simulink model "Complete_System"  (R2018b)
settings: Solver=ode4  StartTime=0.0  StopTime=5  FixedStep=Step_Size  RelTol=1e-3  EnableMultiTasking=on
InitFcn:
  | clc ;
  | clear all ;
  | close all ;
  | Missile_Data ;
  | Sim_Parameters ;
undefined symbols (not defined in the file): D, Tbl_ALPHAT, Tbl_CL_ALPHAT, Tbl_CL_DEL_R, Tbl_CL_P, Tbl_CM_0, Tbl_CM_DEL_P, Tbl_CM_PHIT, Tbl_CM_Q, Tbl_CN_DEL_Y, Tbl_CN_PHIT, Tbl_CN_R, Tbl_CX_0, Tbl_CX_ALPHAT, Tbl_CX_DEL_EFF, Tbl_CY_DEL_Y, Tbl_CY_PHIT, Tbl_CZ_0, Tbl_CZ_DEL_P, Tbl_CZ_PHIT, Tbl_MACH, XCG, XREF
libraries: simulink_extras x4, aerolibtransform2 x3
settings Model: Creator=e803534  LastModifiedBy=auten
settings OptimizationCC: LifeSpan=inf
settings DebuggingCC: UnconnectedInputMsg=none  UnconnectedOutputMsg=none  UnconnectedLineMsg=none  SFUnexpectedBacktrackingDiag=warning  SFNoUnconditionalDefaultTransitionDiag=warning
settings SFSimCC: SimUseLocalCustomCode=off
settings RTWCC: RTWUseLocalCustomCode=off
settings CodeAppCC: StateflowObjectComments=on
settings GRTTargetCC: TargetLangStandard=C89/C90 (ANSI)  GeneratePreprocessorConditionals=Disable all
settings ConfigComp: CovMetricSettings=dw  CovHtmlReporting=on  CovSaveCumulativeToWorkspaceVar=on  CovSaveSingleToWorkspaceVar=on  CovExternalEMLEnable=off

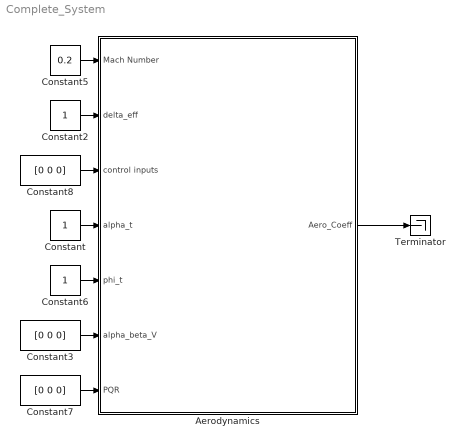
== system Complete_System ==
  Aerodynamics : Subsystem
  Constant : Constant
  Constant2 : Constant
  Constant3 : Constant  Value=[0 0 0]
  Constant5 : Constant  Value=0.2
  Constant6 : Constant
  Constant7 : Constant  Value=[0 0 0]
  Constant8 : Constant  Value=[0 0 0]
  Terminator : Terminator
  wires:
  Constant6/1 -> Aerodynamics/5(phi_t)
  Constant5/1 -> Aerodynamics/1(Mach Number)
  Constant2/1 -> Aerodynamics/2(delta_eff)
  Constant7/1 -> Aerodynamics/7(PQR)
  Constant/1 -> Aerodynamics/4(alpha_t)
  Constant8/1 -> Aerodynamics/3(control inputs)
  Constant3/1 -> Aerodynamics/6(alpha_beta_V)
  Aerodynamics/1(Aero_Coeff) -> Terminator/1

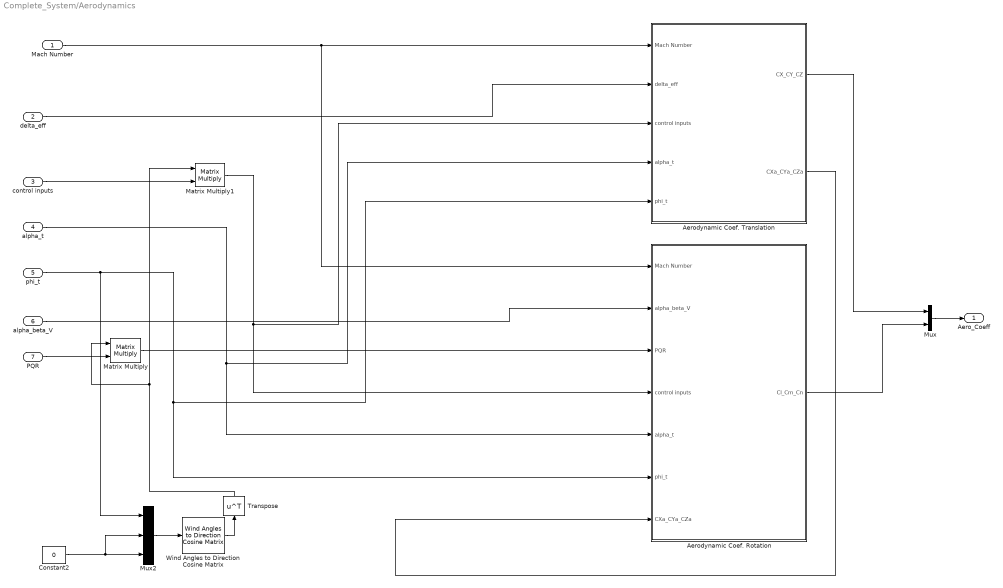
== system Complete_System/Aerodynamics ==
  Mach Number : Inport
  delta_eff : Inport  Port=2
  control inputs : Inport  Port=3
  alpha_t : Inport  Port=4
  phi_t : Inport  Port=5
  alpha_beta_V : Inport  Port=6
  PQR : Inport  Port=7
  Aerodynamic Coef. Rotation : Subsystem
  Aerodynamic Coef. Translation : Subsystem
  Constant2 : Constant  Value=0
  Matrix Multiply : Product  Multiplication=Matrix(*)
  Matrix Multiply1 : Product  Multiplication=Matrix(*)
  Mux : Mux  Inputs=2
  Mux2 : Mux  Inputs=3
  Transpose : Math  Operator=transpose  SaturateOnIntegerOverflow=on
  Wind Angles to Direction Cosine Matrix : aerolibtransform2/Wind Angles to  Direction Cosine Matrix
      settings: SourceProductName=Aerospace Blockset  SourceProductBaseCode=AE
  Aero_Coeff : Outport
  wires:
  Aerodynamic Coef. Translation/2(CXa_CYa_CZa) -> Aerodynamic Coef. Rotation/7(CXa_CYa_CZa)
  Mach Number/1 -> Aerodynamic Coef. Rotation/1(Mach Number), Aerodynamic Coef. Translation/1(Mach Number)
  delta_eff/1 -> Aerodynamic Coef. Translation/2(delta_eff)
  Matrix Multiply1/1 -> Aerodynamic Coef. Rotation/4(control inputs), Aerodynamic Coef. Translation/3(control inputs)
  alpha_beta_V/1 -> Aerodynamic Coef. Rotation/2(alpha_beta_V)
  Matrix Multiply/1 -> Aerodynamic Coef. Rotation/3(PQR)
  Aerodynamic Coef. Translation/1(CX_CY_CZ) -> Mux/1
  Aerodynamic Coef. Rotation/1(Cl_Cm_Cn) -> Mux/2
  Mux/1 -> Aero_Coeff/1
  alpha_t/1 -> Aerodynamic Coef. Rotation/5(alpha_t), Aerodynamic Coef. Translation/4(alpha_t)
  phi_t/1 -> Mux2/1, Aerodynamic Coef. Translation/5(phi_t), Aerodynamic Coef. Rotation/6(phi_t)
  Mux2/1 -> Wind Angles to Direction Cosine Matrix/1
  Constant2/1 -> Mux2/2, Mux2/3
  control inputs/1 -> Matrix Multiply1/2
  Wind Angles to Direction Cosine Matrix/1 -> Transpose/1
  PQR/1 -> Matrix Multiply/2
  Transpose/1 -> Matrix Multiply/1, Matrix Multiply1/1

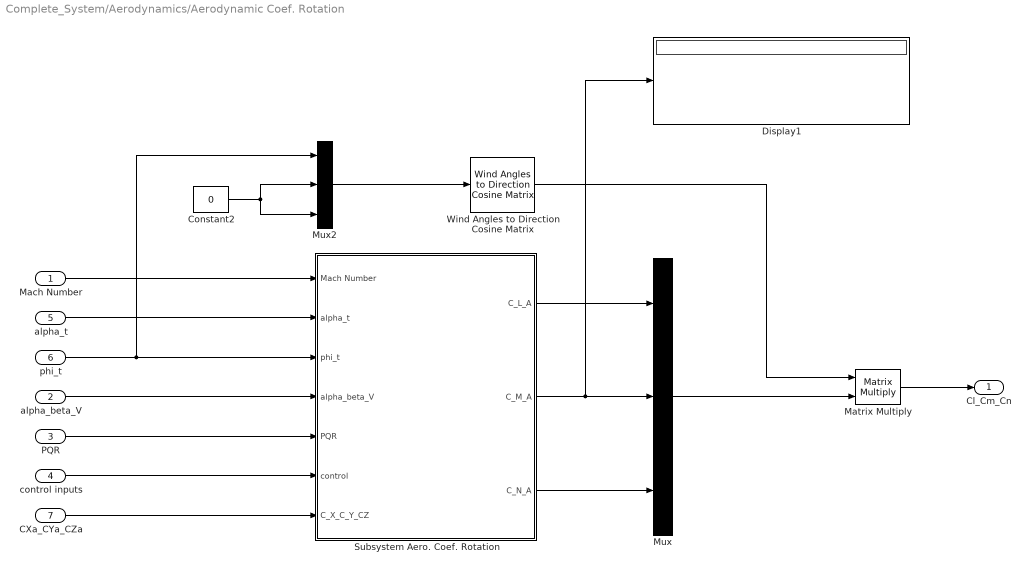
== system Complete_System/Aerodynamics/Aerodynamic Coef. Rotation ==
  Mach Number : Inport
  alpha_beta_V : Inport  Port=2
  PQR : Inport  Port=3
  control inputs : Inport  Port=4
  alpha_t : Inport  Port=5
  phi_t : Inport  Port=6
  CXa_CYa_CZa : Inport  Port=7
  Constant2 : Constant  Value=0
  Display1 : Display
  Matrix Multiply : Product  Multiplication=Matrix(*)
  Mux : Mux  Inputs=3
  Mux2 : Mux  Inputs=3
  Subsystem Aero. Coef. Rotation : Subsystem
  Wind Angles to Direction Cosine Matrix : aerolibtransform2/Wind Angles to  Direction Cosine Matrix
      settings: SourceProductName=Aerospace Blockset  SourceProductBaseCode=AE
  Cl_Cm_Cn : Outport
  wires:
  Mux/1 -> Matrix Multiply/2
  Matrix Multiply/1 -> Cl_Cm_Cn/1
  Mach Number/1 -> Subsystem Aero. Coef. Rotation/1(Mach Number)
  alpha_beta_V/1 -> Subsystem Aero. Coef. Rotation/4(alpha_beta_V)
  PQR/1 -> Subsystem Aero. Coef. Rotation/5(PQR)
  control inputs/1 -> Subsystem Aero. Coef. Rotation/6(control)
  alpha_t/1 -> Subsystem Aero. Coef. Rotation/2(alpha_t)
  phi_t/1 -> Mux2/1, Subsystem Aero. Coef. Rotation/3(phi_t)
  CXa_CYa_CZa/1 -> Subsystem Aero. Coef. Rotation/7(C_X_C_Y_CZ)
  Mux2/1 -> Wind Angles to Direction Cosine Matrix/1
  Constant2/1 -> Mux2/2, Mux2/3
  Wind Angles to Direction Cosine Matrix/1 -> Matrix Multiply/1
  Subsystem Aero. Coef. Rotation/1(C_L_A) -> Mux/1
  Subsystem Aero. Coef. Rotation/2(C_M_A) -> Display1/1, Mux/2
  Subsystem Aero. Coef. Rotation/3(C_N_A) -> Mux/3

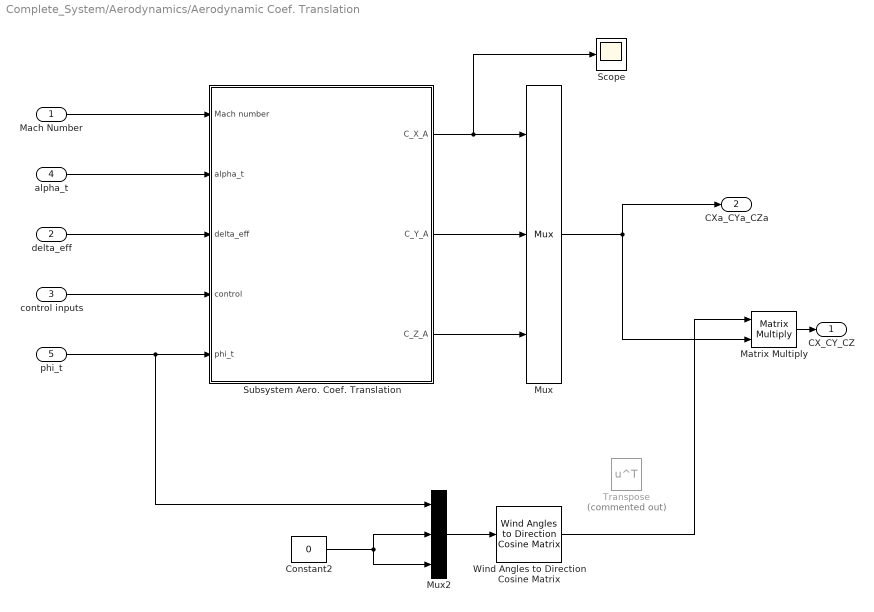
== system Complete_System/Aerodynamics/Aerodynamic Coef. Translation ==
  Mach Number : Inport
  delta_eff : Inport  Port=2
  control inputs : Inport  Port=3
  alpha_t : Inport  Port=4
  phi_t : Inport  Port=5
  Constant2 : Constant  Value=0
  Matrix Multiply : Product  Multiplication=Matrix(*)
  Mux : Mux  Inputs=3
  Mux2 : Mux  Inputs=3
  Scope : Scope
  Subsystem Aero. Coef. Translation : Subsystem
  Transpose : Math  Commented=on  Operator=transpose  SaturateOnIntegerOverflow=on
  Wind Angles to Direction Cosine Matrix : aerolibtransform2/Wind Angles to  Direction Cosine Matrix
      settings: SourceProductName=Aerospace Blockset  SourceProductBaseCode=AE
  CX_CY_CZ : Outport
  CXa_CYa_CZa : Outport  Port=2
  wires:
  Mux/1 -> Matrix Multiply/2, CXa_CYa_CZa/1
  Matrix Multiply/1 -> CX_CY_CZ/1
  Mux2/1 -> Wind Angles to Direction Cosine Matrix/1
  phi_t/1 -> Mux2/1, Subsystem Aero. Coef. Translation/5(phi_t)
  Constant2/1 -> Mux2/2, Mux2/3
  Mach Number/1 -> Subsystem Aero. Coef. Translation/1(Mach number)
  control inputs/1 -> Subsystem Aero. Coef. Translation/4(control)
  alpha_t/1 -> Subsystem Aero. Coef. Translation/2(alpha_t)
  delta_eff/1 -> Subsystem Aero. Coef. Translation/3(delta_eff)
  Subsystem Aero. Coef. Translation/1(C_X_A) -> Scope/1, Mux/1
  Subsystem Aero. Coef. Translation/2(C_Y_A) -> Mux/2
  Subsystem Aero. Coef. Translation/3(C_Z_A) -> Mux/3
  Wind Angles to Direction Cosine Matrix/1 -> Matrix Multiply/1

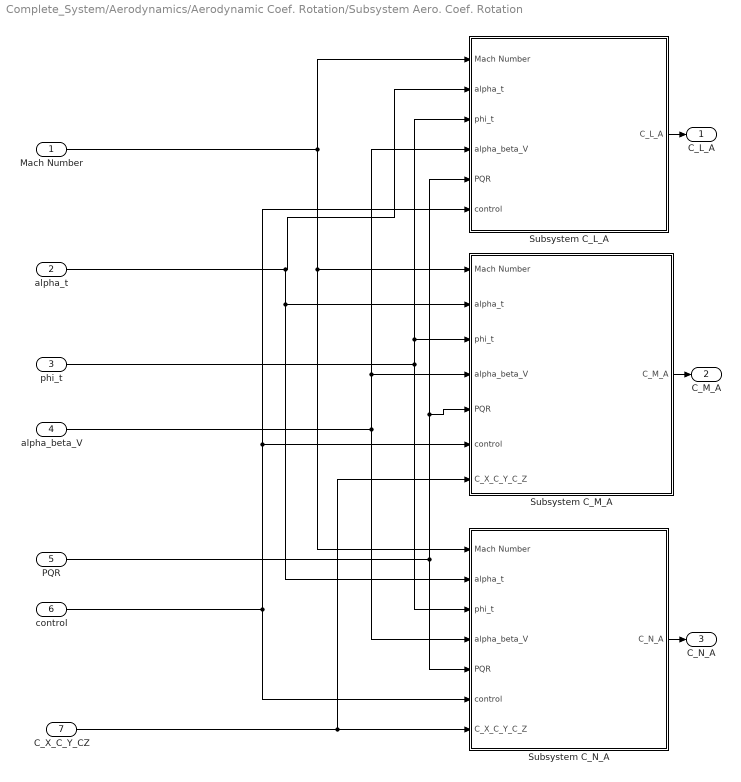
== system Complete_System/Aerodynamics/Aerodynamic Coef. Rotation/Subsystem Aero. Coef. Rotation ==
  Mach Number : Inport
  alpha_t : Inport  Port=2
  phi_t : Inport  Port=3
  alpha_beta_V : Inport  Port=4
  PQR : Inport  Port=5
  control : Inport  Port=6
  C_X_C_Y_CZ : Inport  Port=7
  "Subsystem C_L_A " : Subsystem
  "Subsystem C_M_A " : Subsystem
  Subsystem C_N_A : Subsystem
  C_L_A : Outport
  C_M_A : Outport  Port=2
  C_N_A : Outport  Port=3
  wires:
  "Subsystem C_M_A "/1(C_M_A) -> C_M_A/1
  "Subsystem C_L_A "/1(C_L_A) -> C_L_A/1
  Subsystem C_N_A/1(C_N_A) -> C_N_A/1
  Mach Number/1 -> "Subsystem C_L_A "/1(Mach Number), "Subsystem C_M_A "/1(Mach Number), Subsystem C_N_A/1(Mach Number)
  alpha_t/1 -> Subsystem C_N_A/2(alpha_t), "Subsystem C_M_A "/2(alpha_t), "Subsystem C_L_A "/2(alpha_t)
  phi_t/1 -> Subsystem C_N_A/3(phi_t), "Subsystem C_M_A "/3(phi_t), "Subsystem C_L_A "/3(phi_t)
  alpha_beta_V/1 -> "Subsystem C_L_A "/4(alpha_beta_V), "Subsystem C_M_A "/4(alpha_beta_V), Subsystem C_N_A/4(alpha_beta_V)
  PQR/1 -> "Subsystem C_M_A "/5(PQR), "Subsystem C_L_A "/5(PQR), Subsystem C_N_A/5(PQR)
  control/1 -> "Subsystem C_M_A "/6(control), "Subsystem C_L_A "/6(control), Subsystem C_N_A/6(control)
  C_X_C_Y_CZ/1 -> "Subsystem C_M_A "/7(C_X_C_Y_C_Z), Subsystem C_N_A/7(C_X_C_Y_C_Z)

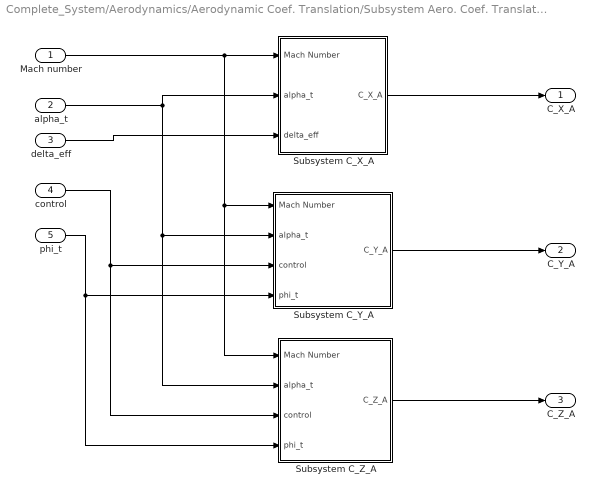
== system Complete_System/Aerodynamics/Aerodynamic Coef. Translation/Subsystem Aero. Coef. Translation ==
  Mach number : Inport
  alpha_t : Inport  Port=2
  delta_eff : Inport  Port=3
  control : Inport  Port=4
  phi_t : Inport  Port=5
  Subsystem C_X_A : Subsystem
  Subsystem C_Y_A : Subsystem
  Subsystem C_Z_A : Subsystem
  C_X_A : Outport
  C_Y_A : Outport  Port=2
  C_Z_A : Outport  Port=3
  wires:
  Subsystem C_X_A/1(C_X_A) -> C_X_A/1
  Subsystem C_Y_A/1(C_Y_A) -> C_Y_A/1
  Subsystem C_Z_A/1(C_Z_A) -> C_Z_A/1
  Mach number/1 -> Subsystem C_Z_A/1(Mach Number), Subsystem C_Y_A/1(Mach Number), Subsystem C_X_A/1(Mach Number)
  alpha_t/1 -> Subsystem C_Z_A/2(alpha_t), Subsystem C_Y_A/2(alpha_t), Subsystem C_X_A/2(alpha_t)
  delta_eff/1 -> Subsystem C_X_A/3(delta_eff)
  control/1 -> Subsystem C_Z_A/3(control), Subsystem C_Y_A/3(control)
  phi_t/1 -> Subsystem C_Z_A/4(phi_t), Subsystem C_Y_A/4(phi_t)

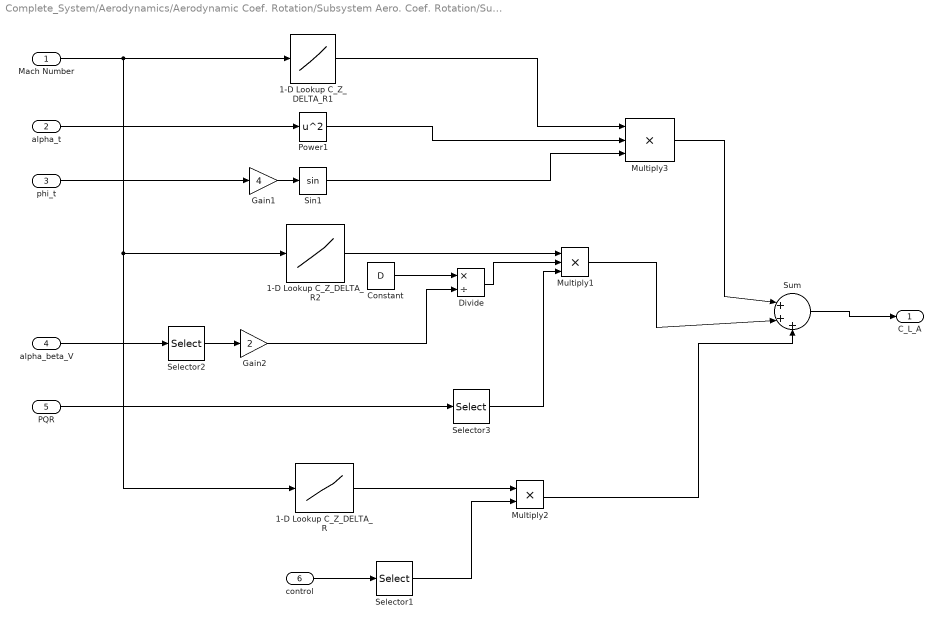
== system Complete_System/Aerodynamics/Aerodynamic Coef. Rotation/Subsystem Aero. Coef. Rotation/Subsystem C_L_A  ==
  Mach Number : Inport
  alpha_t : Inport  Port=2
  phi_t : Inport  Port=3
  alpha_beta_V : Inport  Port=4
  PQR : Inport  Port=5
  control : Inport  Port=6
  1-D Lookup C_Z_DELTA_R : Lookup_n-D  NumberOfTableDimensions=1  BreakpointsForDimension1=Tbl_MACH  Table=Tbl_CL_DEL_R  InternalRulePriority=Speed  RndMeth=Simplest  InputSameDT=on
  1-D Lookup C_Z_DELTA_R1 : Lookup_n-D  NumberOfTableDimensions=1  BreakpointsForDimension1=Tbl_MACH  Table=Tbl_CL_ALPHAT  InternalRulePriority=Speed  RndMeth=Simplest  InputSameDT=on
  1-D Lookup C_Z_DELTA_R2 : Lookup_n-D  NumberOfTableDimensions=1  BreakpointsForDimension1=Tbl_MACH  Table=Tbl_CL_P  InternalRulePriority=Speed  RndMeth=Simplest  InputSameDT=on
  Constant : Constant  Value=D
  Divide : Product  Inputs=*/
  Gain1 : Gain  Gain=4
  Gain2 : Gain  Gain=2
  Multiply1 : Product  Inputs=3
  Multiply2 : Product
  Multiply3 : Product  Inputs=3
  Power1 : Math  Operator=square  SaturateOnIntegerOverflow=on
  Selector1 : Selector  InputPortWidth=3  IndexOptions=Index vector (dialog)  Indices=[1]  OutputSizes=1
  Selector2 : Selector  InputPortWidth=3  IndexOptions=Index vector (dialog)  Indices=[3]  OutputSizes=1
  Selector3 : Selector  InputPortWidth=3  IndexOptions=Index vector (dialog)  Indices=[1]  OutputSizes=1
  Sin1 : Trigonometry
  Sum : Sum  Inputs=|+++
  C_L_A : Outport
  wires:
  1-D Lookup C_Z_DELTA_R1/1 -> Multiply3/1
  alpha_t/1 -> Power1/1
  Sum/1 -> C_L_A/1
  Mach Number/1 -> 1-D Lookup C_Z_DELTA_R/1, 1-D Lookup C_Z_DELTA_R2/1, 1-D Lookup C_Z_DELTA_R1/1
  1-D Lookup C_Z_DELTA_R2/1 -> Multiply1/1
  1-D Lookup C_Z_DELTA_R/1 -> Multiply2/1
  Multiply2/1 -> Sum/3
  Power1/1 -> Multiply3/2
  Sin1/1 -> Multiply3/3
  phi_t/1 -> Gain1/1
  Gain1/1 -> Sin1/1
  alpha_beta_V/1 -> Selector2/1
  Multiply3/1 -> Sum/1
  Multiply1/1 -> Sum/2
  Constant/1 -> Divide/1
  Selector2/1 -> Gain2/1
  Gain2/1 -> Divide/2
  Divide/1 -> Multiply1/2
  PQR/1 -> Selector3/1
  Selector3/1 -> Multiply1/3
  control/1 -> Selector1/1
  Selector1/1 -> Multiply2/2

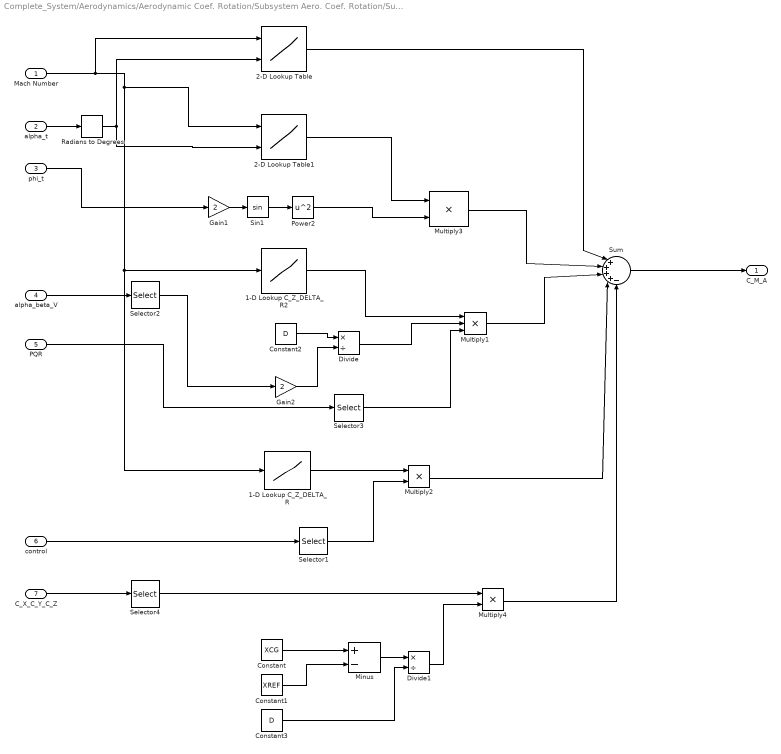
== system Complete_System/Aerodynamics/Aerodynamic Coef. Rotation/Subsystem Aero. Coef. Rotation/Subsystem C_M_A  ==
  Mach Number : Inport
  alpha_t : Inport  Port=2
  phi_t : Inport  Port=3
  alpha_beta_V : Inport  Port=4
  PQR : Inport  Port=5
  control : Inport  Port=6
  C_X_C_Y_C_Z : Inport  Port=7
  1-D Lookup C_Z_DELTA_R : Lookup_n-D  NumberOfTableDimensions=1  BreakpointsForDimension1=Tbl_MACH  Table=Tbl_CM_DEL_P  InternalRulePriority=Speed  RndMeth=Simplest  InputSameDT=on
  1-D Lookup C_Z_DELTA_R2 : Lookup_n-D  NumberOfTableDimensions=1  BreakpointsForDimension1=Tbl_MACH  Table=Tbl_CM_Q  DiagnosticForOutOfRangeInput=Warning  InternalRulePriority=Speed  RndMeth=Simplest  InputSameDT=on
  2-D Lookup Table : Lookup_n-D  BreakpointsForDimension1=Tbl_MACH  BreakpointsForDimension2=Tbl_ALPHAT  Table=Tbl_CM_0  DiagnosticForOutOfRangeInput=Warning  InternalRulePriority=Speed  RndMeth=Simplest  InputSameDT=on
  2-D Lookup Table1 : Lookup_n-D  BreakpointsForDimension1=Tbl_MACH  BreakpointsForDimension2=Tbl_ALPHAT  Table=Tbl_CM_PHIT  InternalRulePriority=Speed  RndMeth=Simplest  InputSameDT=on
  Constant : Constant  Value=XCG
  Constant1 : Constant  Value=XREF
  Constant2 : Constant  Value=D
  Constant3 : Constant  Value=D
  Divide : Product  Inputs=*/
  Divide1 : Product  Inputs=*/
  Gain1 : Gain  Gain=2
  Gain2 : Gain  Gain=2
  Minus : Sum  Inputs=+-
  Multiply1 : Product  Inputs=3
  Multiply2 : Product
  Multiply3 : Product
  Multiply4 : Product
  Power2 : Math  Operator=square  SaturateOnIntegerOverflow=on
  Radians to Degrees : simulink_extras/Transformations/Radians to Degrees
  Selector1 : Selector  InputPortWidth=3  IndexOptions=Index vector (dialog)  Indices=[2]  OutputSizes=1
  Selector2 : Selector  InputPortWidth=3  IndexOptions=Index vector (dialog)  Indices=[3]  OutputSizes=1
  Selector3 : Selector  InputPortWidth=3  IndexOptions=Index vector (dialog)  Indices=[2]  OutputSizes=1
  Selector4 : Selector  InputPortWidth=3  IndexOptions=Index vector (dialog)  Indices=[3]  OutputSizes=1
  Sin1 : Trigonometry
  Sum : Sum  Inputs=|++++-
  C_M_A : Outport
  wires:
  2-D Lookup Table/1 -> Sum/1
  Mach Number/1 -> 2-D Lookup Table/1, 2-D Lookup Table1/1, 1-D Lookup C_Z_DELTA_R/1, 1-D Lookup C_Z_DELTA_R2/1
  1-D Lookup C_Z_DELTA_R2/1 -> Multiply1/1
  1-D Lookup C_Z_DELTA_R/1 -> Multiply2/1
  Multiply2/1 -> Sum/4
  Sin1/1 -> Power2/1
  phi_t/1 -> Gain1/1
  Gain1/1 -> Sin1/1
  alpha_beta_V/1 -> Selector2/1
  Selector2/1 -> Gain2/1
  Gain2/1 -> Divide/2
  Divide/1 -> Multiply1/2
  PQR/1 -> Selector3/1
  Selector3/1 -> Multiply1/3
  control/1 -> Selector1/1
  Selector1/1 -> Multiply2/2
  2-D Lookup Table1/1 -> Multiply3/1
  Power2/1 -> Multiply3/2
  C_X_C_Y_C_Z/1 -> Selector4/1
  Constant/1 -> Minus/1
  Constant1/1 -> Minus/2
  Constant2/1 -> Divide/1
  Minus/1 -> Divide1/1
  Constant3/1 -> Divide1/2
  Selector4/1 -> Multiply4/1
  Divide1/1 -> Multiply4/2
  Multiply4/1 -> Sum/5
  Multiply1/1 -> Sum/3
  Multiply3/1 -> Sum/2
  alpha_t/1 -> Radians to Degrees/1
  Radians to Degrees/1 -> 2-D Lookup Table1/2, 2-D Lookup Table/2
  Sum/1 -> C_M_A/1

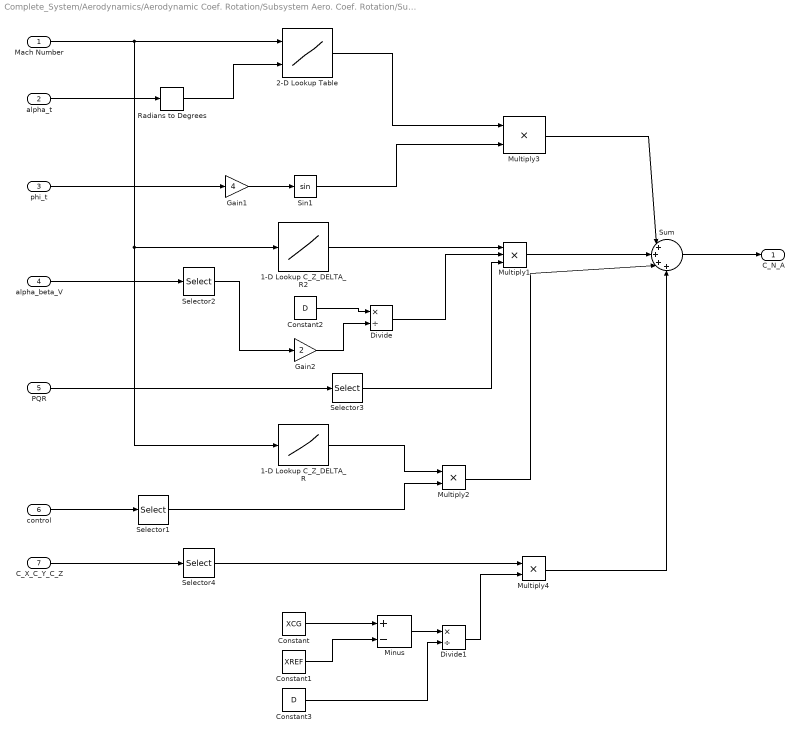
== system Complete_System/Aerodynamics/Aerodynamic Coef. Rotation/Subsystem Aero. Coef. Rotation/Subsystem C_N_A ==
  Mach Number : Inport
  alpha_t : Inport  Port=2
  phi_t : Inport  Port=3
  alpha_beta_V : Inport  Port=4
  PQR : Inport  Port=5
  control : Inport  Port=6
  C_X_C_Y_C_Z : Inport  Port=7
  1-D Lookup C_Z_DELTA_R : Lookup_n-D  NumberOfTableDimensions=1  BreakpointsForDimension1=Tbl_MACH  Table=Tbl_CN_DEL_Y  InternalRulePriority=Speed  RndMeth=Simplest  InputSameDT=on
  1-D Lookup C_Z_DELTA_R2 : Lookup_n-D  NumberOfTableDimensions=1  BreakpointsForDimension1=Tbl_MACH  Table=Tbl_CN_R  InternalRulePriority=Speed  RndMeth=Simplest  InputSameDT=on
  2-D Lookup Table : Lookup_n-D  BreakpointsForDimension1=Tbl_MACH  BreakpointsForDimension2=Tbl_ALPHAT  Table=Tbl_CN_PHIT  InternalRulePriority=Speed  RndMeth=Simplest  InputSameDT=on
  Constant : Constant  Value=XCG
  Constant1 : Constant  Value=XREF
  Constant2 : Constant  Value=D
  Constant3 : Constant  Value=D
  Divide : Product  Inputs=*/
  Divide1 : Product  Inputs=*/
  Gain1 : Gain  Gain=4
  Gain2 : Gain  Gain=2
  Minus : Sum  Inputs=+-
  Multiply1 : Product  Inputs=3
  Multiply2 : Product
  Multiply3 : Product
  Multiply4 : Product
  Radians to Degrees : simulink_extras/Transformations/Radians to Degrees
  Selector1 : Selector  InputPortWidth=3  IndexOptions=Index vector (dialog)  Indices=[3]  OutputSizes=1
  Selector2 : Selector  InputPortWidth=3  IndexOptions=Index vector (dialog)  Indices=[3]  OutputSizes=1
  Selector3 : Selector  InputPortWidth=3  IndexOptions=Index vector (dialog)  Indices=[3]  OutputSizes=1
  Selector4 : Selector  InputPortWidth=3  IndexOptions=Index vector (dialog)  Indices=[2]  OutputSizes=1
  Sin1 : Trigonometry
  Sum : Sum  Inputs=|++++
  C_N_A : Outport
  wires:
  2-D Lookup Table/1 -> Multiply3/1
  alpha_t/1 -> Radians to Degrees/1
  Sum/1 -> C_N_A/1
  Mach Number/1 -> 2-D Lookup Table/1, 1-D Lookup C_Z_DELTA_R/1, 1-D Lookup C_Z_DELTA_R2/1
  1-D Lookup C_Z_DELTA_R2/1 -> Multiply1/1
  1-D Lookup C_Z_DELTA_R/1 -> Multiply2/1
  Multiply2/1 -> Sum/3
  Sin1/1 -> Multiply3/2
  phi_t/1 -> Gain1/1
  Gain1/1 -> Sin1/1
  alpha_beta_V/1 -> Selector2/1
  Selector2/1 -> Gain2/1
  Divide/1 -> Multiply1/2
  PQR/1 -> Selector3/1
  Selector3/1 -> Multiply1/3
  control/1 -> Selector1/1
  Selector1/1 -> Multiply2/2
  C_X_C_Y_C_Z/1 -> Selector4/1
  Constant/1 -> Minus/1
  Constant1/1 -> Minus/2
  Constant2/1 -> Divide/1
  Minus/1 -> Divide1/1
  Constant3/1 -> Divide1/2
  Selector4/1 -> Multiply4/1
  Divide1/1 -> Multiply4/2
  Multiply4/1 -> Sum/4
  Multiply1/1 -> Sum/2
  Multiply3/1 -> Sum/1
  Radians to Degrees/1 -> 2-D Lookup Table/2
  Gain2/1 -> Divide/2

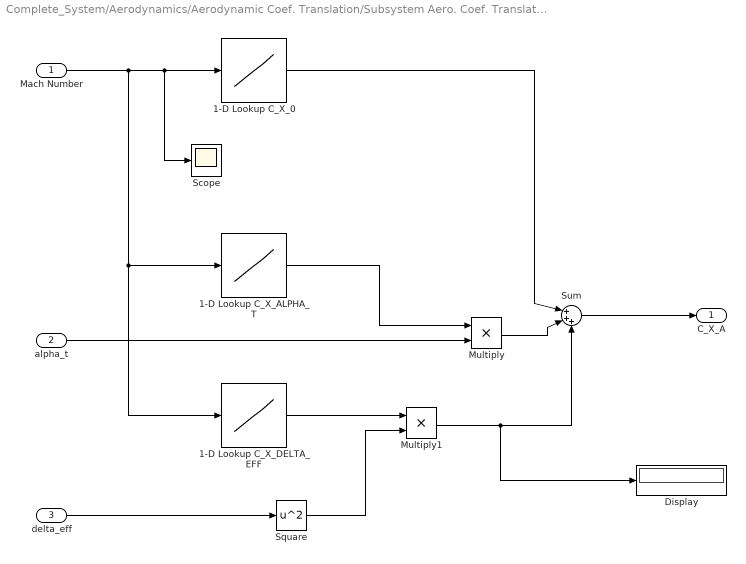
== system Complete_System/Aerodynamics/Aerodynamic Coef. Translation/Subsystem Aero. Coef. Translation/Subsystem C_X_A ==
  Mach Number : Inport
  alpha_t : Inport  Port=2
  delta_eff : Inport  Port=3
  1-D Lookup C_X_0 : Lookup_n-D  NumberOfTableDimensions=1  BreakpointsForDimension1=Tbl_MACH  Table=Tbl_CX_0  DiagnosticForOutOfRangeInput=Error  InternalRulePriority=Speed  RndMeth=Simplest  InputSameDT=on
  1-D Lookup C_X_ALPHA_T : Lookup_n-D  NumberOfTableDimensions=1  BreakpointsForDimension1=Tbl_MACH  BeginIndexSearchUsingPreviousIndexResult=on  Table=Tbl_CX_ALPHAT  DiagnosticForOutOfRangeInput=Error  InternalRulePriority=Speed  RndMeth=Simplest  InputSameDT=on
  1-D Lookup C_X_DELTA_EFF : Lookup_n-D  NumberOfTableDimensions=1  BreakpointsForDimension1=Tbl_MACH  Table=Tbl_CX_DEL_EFF  DiagnosticForOutOfRangeInput=Error  InternalRulePriority=Speed  RndMeth=Simplest  InputSameDT=on
  Display : Display
  Multiply : Product
  Multiply1 : Product
  Scope : Scope
  Square : Math  Operator=square  SaturateOnIntegerOverflow=on
  Sum : Sum  Inputs=|+++
  C_X_A : Outport
  wires:
  Multiply/1 -> Sum/2
  Multiply1/1 -> Display/1, Sum/3
  1-D Lookup C_X_DELTA_EFF/1 -> Multiply1/1
  1-D Lookup C_X_ALPHA_T/1 -> Multiply/1
  1-D Lookup C_X_0/1 -> Sum/1
  Mach Number/1 -> 1-D Lookup C_X_DELTA_EFF/1, 1-D Lookup C_X_ALPHA_T/1, Scope/1, 1-D Lookup C_X_0/1
  Sum/1 -> C_X_A/1
  alpha_t/1 -> Multiply/2
  delta_eff/1 -> Square/1
  Square/1 -> Multiply1/2

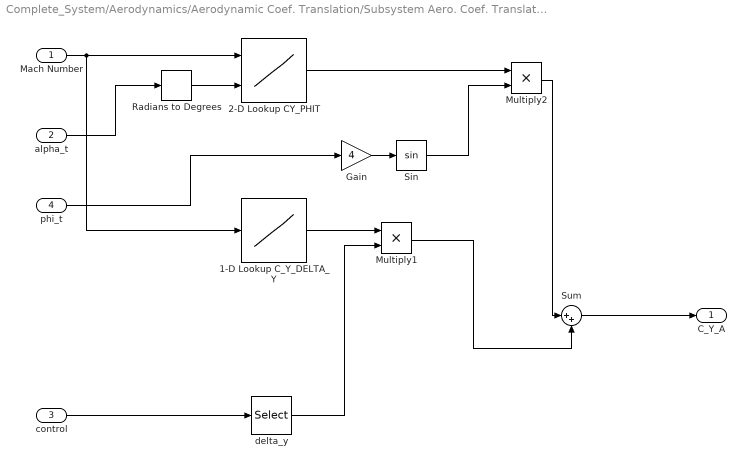
== system Complete_System/Aerodynamics/Aerodynamic Coef. Translation/Subsystem Aero. Coef. Translation/Subsystem C_Y_A ==
  Mach Number : Inport
  alpha_t : Inport  Port=2
  control : Inport  Port=3
  phi_t : Inport  Port=4
  1-D Lookup C_Y_DELTA_Y : Lookup_n-D  NumberOfTableDimensions=1  BreakpointsForDimension1=Tbl_MACH  Table=Tbl_CY_DEL_Y  InternalRulePriority=Speed  RndMeth=Simplest  InputSameDT=on
  2-D Lookup CY_PHIT : Lookup_n-D  BreakpointsForDimension1=Tbl_MACH  BreakpointsForDimension2=Tbl_ALPHAT  Table=Tbl_CY_PHIT  InternalRulePriority=Speed  RndMeth=Simplest  InputSameDT=on
  Gain : Gain  Gain=4
  Multiply1 : Product
  Multiply2 : Product
  Radians to Degrees : simulink_extras/Transformations/Radians to Degrees
  Sin : Trigonometry
  Sum : Sum  Inputs=|++
  delta_y : Selector  InputPortWidth=3  IndexOptions=Index vector (dialog)  Indices=[3]  OutputSizes=1
  C_Y_A : Outport
  wires:
  Multiply1/1 -> Sum/2
  1-D Lookup C_Y_DELTA_Y/1 -> Multiply1/1
  2-D Lookup CY_PHIT/1 -> Multiply2/1
  Mach Number/1 -> 1-D Lookup C_Y_DELTA_Y/1, 2-D Lookup CY_PHIT/1
  Sum/1 -> C_Y_A/1
  Gain/1 -> Sin/1
  phi_t/1 -> Gain/1
  control/1 -> delta_y/1
  alpha_t/1 -> Radians to Degrees/1
  delta_y/1 -> Multiply1/2
  Sin/1 -> Multiply2/2
  Multiply2/1 -> Sum/1
  Radians to Degrees/1 -> 2-D Lookup CY_PHIT/2

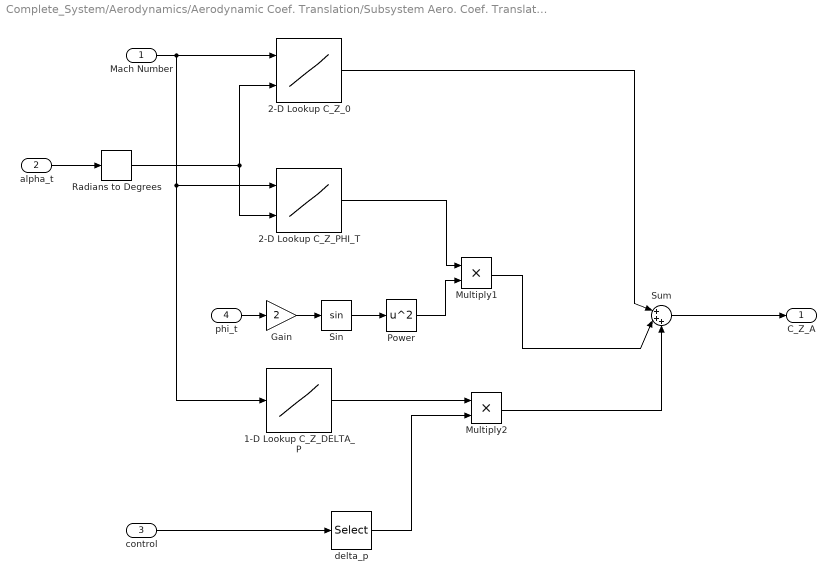
== system Complete_System/Aerodynamics/Aerodynamic Coef. Translation/Subsystem Aero. Coef. Translation/Subsystem C_Z_A ==
  Mach Number : Inport
  alpha_t : Inport  Port=2
  control : Inport  Port=3
  phi_t : Inport  Port=4
  1-D Lookup C_Z_DELTA_P : Lookup_n-D  NumberOfTableDimensions=1  BreakpointsForDimension1=Tbl_MACH  Table=Tbl_CZ_DEL_P  InternalRulePriority=Speed  RndMeth=Simplest  InputSameDT=on
  2-D Lookup C_Z_0 : Lookup_n-D  BreakpointsForDimension1=Tbl_MACH  BreakpointsForDimension2=Tbl_ALPHAT  Table=Tbl_CZ_0  DiagnosticForOutOfRangeInput=Warning  InternalRulePriority=Speed  RndMeth=Simplest  InputSameDT=on
  2-D Lookup C_Z_PHI_T : Lookup_n-D  BreakpointsForDimension1=Tbl_MACH  BreakpointsForDimension2=Tbl_ALPHAT  Table=Tbl_CZ_PHIT  InternalRulePriority=Speed  RndMeth=Simplest  InputSameDT=on
  Gain : Gain  Gain=2
  Multiply1 : Product
  Multiply2 : Product
  Power : Math  Operator=square  SaturateOnIntegerOverflow=on
  Radians to Degrees : simulink_extras/Transformations/Radians to Degrees
  Sin : Trigonometry
  Sum : Sum  Inputs=|+++
  delta_p : Selector  InputPortWidth=3  IndexOptions=Index vector (dialog)  Indices=[2]  OutputSizes=1
  C_Z_A : Outport
  wires:
  2-D Lookup C_Z_0/1 -> Sum/1
  delta_p/1 -> Multiply2/2
  alpha_t/1 -> Radians to Degrees/1
  control/1 -> delta_p/1
  Sum/1 -> C_Z_A/1
  Mach Number/1 -> 2-D Lookup C_Z_PHI_T/1, 1-D Lookup C_Z_DELTA_P/1, 2-D Lookup C_Z_0/1
  2-D Lookup C_Z_PHI_T/1 -> Multiply1/1
  Multiply1/1 -> Sum/2
  Gain/1 -> Sin/1
  phi_t/1 -> Gain/1
  Sin/1 -> Power/1
  Power/1 -> Multiply1/2
  1-D Lookup C_Z_DELTA_P/1 -> Multiply2/1
  Multiply2/1 -> Sum/3
  Radians to Degrees/1 -> 2-D Lookup C_Z_0/2, 2-D Lookup C_Z_PHI_T/2
